simulink model "LMSzero"  (R2015b)
settings: Solver=VariableStepAuto  StartTime=0.0  StopTime=inf  RelTol=1e-3
libraries: dspsrcs4 x1, dspadpt3 x1, dspsnks4 x1
settings Model: Creator=User  LastModifiedBy=Chao

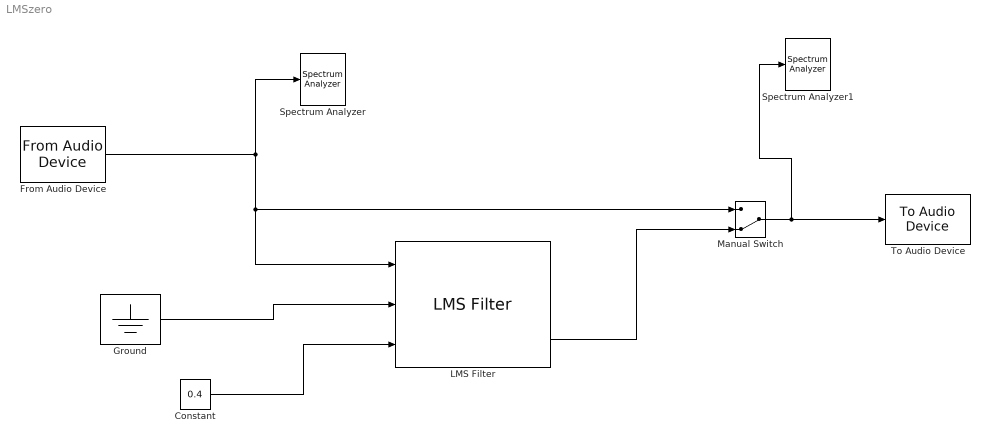
== system LMSzero ==
  Constant : Constant  Value=0.4
  From Audio Device : dspsrcs4/From Audio Device  deviceName=Default  numChannels=1  sampleRate=44100  deviceDatatype=Determine from output data type  autoBufferSize=on  bufferSize=4096  queueDuration=1.0  frameSize=1024  outputDatatype=double  defaultInputChannelMapping=on  inputChannelMapping=1:2  outputNumOverrunSamples=off  OutputFrames=off
  Ground : Ground
  LMS Filter : dspadpt3/LMS Filter  Algo=LMS  L=40  stepflag=Input port  mu=0.1  leakage=1.0  ic=0  Adapt=off  resetflag=None  weights=off  secondCoeffMode=User-defined  secondCoeffWordLength=2  secondCoeffFracLength=15  accum2Mode=User-defined  accum2FracLength=20  prodOutput2Mode=User-defined  prodOutput2FracLength=20  prodOutput3Mode=User-defined  prodOutput3FracLength=20  prodOutput4Mode=User-defined  prodOutput4FracLength=20  quotientMode=User-defined  quotientFracLength=20  roundingMode=Floor  overflowMode=off  addnparflag=off
  Manual Switch : ManualSwitch  CurrentSetting=0
  Spectrum Analyzer : SpectrumAnalyzer
  Spectrum Analyzer1 : SpectrumAnalyzer
  To Audio Device : dspsnks4/To Audio Device  deviceName=Default  inheritSampleRate=on  sampleRate=44100  deviceDatatype=Determine from input data type  autoBufferSize=on  bufferSize=4096  queueDuration=1.0  defaultOutputChannelMapping=on  outputChannelMapping=1:2  outputNumUnderrunSamples=off
  wires:
  Ground/1 -> LMS Filter/2
  Constant/1 -> LMS Filter/3
  From Audio Device/1 -> Spectrum Analyzer/1, Manual Switch/1, LMS Filter/1
  Manual Switch/1 -> Spectrum Analyzer1/1, To Audio Device/1
  LMS Filter/2 -> Manual Switch/2
